simulink model "conversion_force_to_attitude"  (R2020a)
settings: Solver=FixedStepAuto  StartTime=0.0  StopTime=10.0  RelTol=1e-3
undefined symbols (not defined in the file): sim_freq
settings Model: Creator=francois  LastModifiedBy=murray

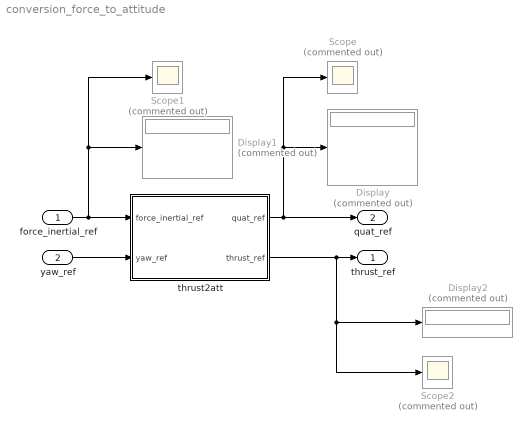
== system conversion_force_to_attitude ==
  force_inertial_ref : Inport
  yaw_ref : Inport  Port=2
  Display : Display  Commented=on
  Display1 : Display  Commented=on
  Display2 : Display  Commented=on
  Scope : Scope  Commented=on
  Scope1 : Scope  Commented=on
  Scope2 : Scope  Commented=on
  thrust2att : MATLAB Function  TreatAsAtomicUnit=on  SystemSampleTime=1/sim_freq
  thrust_ref : Outport  VectorParamsAs1DForOutWhenUnconnected=off
  quat_ref : Outport  Port=2  VectorParamsAs1DForOutWhenUnconnected=off
  wires:
  thrust2att/1(quat_ref) -> Scope/1, Display/1, quat_ref/1
  thrust2att/2(thrust_ref) -> Scope2/1, Display2/1, thrust_ref/1
  yaw_ref/1 -> thrust2att/2(yaw_ref)
  force_inertial_ref/1 -> Scope1/1, Display1/1, thrust2att/1(force_inertial_ref)

== matlab function conversion_force_to_attitude/thrust2att ==
  data: force_inertial_ref input size=3; quat_ref output size=4; yaw_ref input size=1; thrust_ref output size=1
function [quat_ref, thrust_ref] = thrust2att(force_inertial_ref, yaw_ref)
    coder.extrinsic('dcm2quat');

        % Initialise quat
    quat_ref = [1; 0; 0; 0];
    
    % Thrust is norm of force
    thrust_ref = norm(force_inertial_ref);
    
    % Determine body_z rotation (fit body_z onto z axis of force)
    if thrust_ref > 1e-6
        body_z = -force_inertial_ref./thrust_ref;
    else
       body_z = [0; 0; 1]; 
    end
    
    % Determine body_x
    yaw_dir = [-sin(yaw_ref); cos(yaw_ref); 0];
    
    if abs(body_z(3)) > 1e-6
        body_x = cross(yaw_dir, body_z);
        
        if body_z(3) < 0
            body_x = -body_x;
        end
        body_x = body_x ./ norm(body_x);
    else
        body_x = [0; 0; 1];
    end
    
    % Determine body_y
    body_y = cross(body_z, body_x);
    body_y = body_y ./ norm(body_y);
    
    % Calculate rotation
    dcm = [body_x body_y body_z];
    quat_ref = dcm2quat(dcm');
    
    % Normalise quaternion
    quat_ref = quat_ref ./ norm(quat_ref);
    
end
